simulink model "Controller_Model"  (R2015a)
settings: Solver=ode45  StartTime=0.0  StopTime=100.0  RelTol=1e-3
values from neighbouring files (symbols this model uses):
  Hph = tfest(dataPhi, [2 2], [2 2], 'Ts', Te)    [Models.m]    (also in shit_try.m = tfest(dataPhi, [2 2], [2 2], Options); smth_new_025.m = tfest(dataPhi, [6 6], [1 1], Options))
  Hphdot = tfest(dataPHId, 2, 2, 'Ts', Te)    [Models.m]    (also in shit_try.m = tfest(dataPHId, 1, 1, Options); smth_new_025.m = tfest(dataPHId, 2, 1, Options, 'Ts', Te, 'Feedthrough', true)
  Hps = tfest(dataPSI, [2 2], [1 1], 'Ts', Te)    [Models.m]    (also in shit_try.m = tfest(dataPSI, [2 2], [1 1], Options); smth_new_025.m = tfest(dataPSI, [7 7], [1 1], Options))
  Hpsdot = idtf(Hpsdot)    [Models.m]    (also in shit_try.m = tfest(dataPSdot, 1, 1, Options); smth_new_025.m = tfest(dataPSdot, 2, 2, Options, 'Ts', Te, 'Feedthrough', tru)
  Hth = tfest(dataTH, [2 2], [1 1], 'Ts', Te)    [Models.m]    (also in shit_try.m = tfest(dataTH, [2 2], [2 2], Options); smth_new_025.m = tfest(dataTH, [4 4], [4 4], Options))
  Hthdot = idtf(Hthdot)    [Models.m]    (also in shit_try.m = tfest(dataTHdot, 1, 1, Options); smth_new_025.m = tfest(dataTHdot, 2, 2, 'Ts', Te))
  K = lqr(Hf_MIMO.a, Hf_MIMO.b, Q, R)    [Models.m]    (also in shit_try.m)
  Te = t(2)-t(1)    [Models.m]    (also in shit_try.m = 0.003; simData_check.mat = 0.01; smth_new_025.m)
settings Model: Creator=Maria  LastModifiedBy=Maria

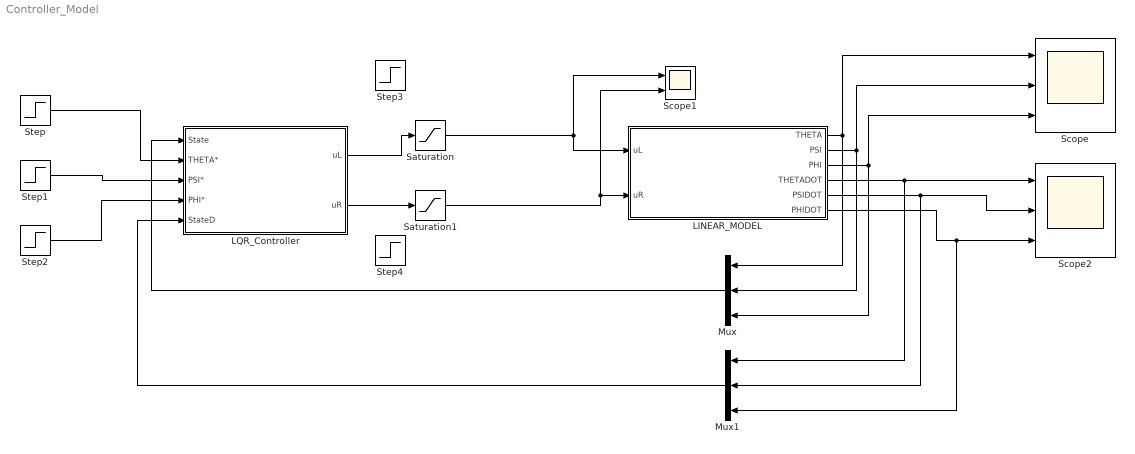
== system Controller_Model ==
  "LINEAR_MODEL " : Subsystem
  "LQR_Controller " : Subsystem
  Mux : Mux  Inputs=3
  Mux1 : Mux  Inputs=3
  Saturation : Saturate  UpperLimit=0.7  LowerLimit=-0.7
  Saturation1 : Saturate  UpperLimit=0.7  LowerLimit=-0.7
  Scope : Scope  NumInputPorts=3
      settings: YMin=-5~-5~-5  YMax=5~5~5
  Scope1 : Scope  NumInputPorts=2
      settings: YMin=-5~-5  YMax=5~5
  Scope2 : Scope  NumInputPorts=3
      settings: YMin=-5~-5~-5  YMax=5~5~5  SaveName=ScopeData2
  Step : Step  Time=0  After=0.01  SampleTime=0
  Step1 : Step  Time=0  After=0  SampleTime=0
  Step2 : Step  Time=0  After=0  SampleTime=0
  Step3 : Step  Time=0  After=0.25  SampleTime=0
  Step4 : Step  Time=0  After=0.25  SampleTime=0
  wires:
  "LINEAR_MODEL "/1("THETA ") -> Scope/1, Mux/1
  "LINEAR_MODEL "/2("PSI ") -> Mux/2, Scope/2
  "LINEAR_MODEL "/3("PHI ") -> Mux/3, Scope/3
  "LINEAR_MODEL "/4("THETADOT ") -> Mux1/1, Scope2/1
  "LINEAR_MODEL "/5("PSIDOT ") -> Scope2/2, Mux1/2
  "LINEAR_MODEL "/6("PHIDOT ") -> Mux1/3, Scope2/3
  Mux/1 -> "LQR_Controller "/1("State ")
  Step/1 -> "LQR_Controller "/2(THETA*)
  Step1/1 -> "LQR_Controller "/3("PSI* ")
  Step2/1 -> "LQR_Controller "/4("PHI* ")
  "LQR_Controller "/1("uL ") -> Saturation/1
  "LQR_Controller "/2("uR ") -> Saturation1/1
  Mux1/1 -> "LQR_Controller "/5("StateD ")
  Saturation/1 -> "LINEAR_MODEL "/1("uL "), Scope1/1
  Saturation1/1 -> Scope1/2, "LINEAR_MODEL "/2("uR ")

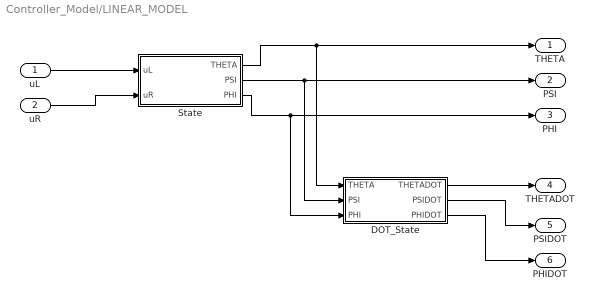
== system Controller_Model/LINEAR_MODEL  ==
  "uL " : Inport
  "uR " : Inport  Port=2
  "DOT_State " : Subsystem
  "State " : Subsystem
  "THETA " : Outport
  "PSI " : Outport  Port=2
  "PHI " : Outport  Port=3
  "THETADOT " : Outport  Port=4
  "PSIDOT " : Outport  Port=5
  "PHIDOT " : Outport  Port=6
  wires:
  "uL "/1 -> "State "/1("uL ")
  "uR "/1 -> "State "/2("uR ")
  "State "/1("THETA ") -> "THETA "/1, "DOT_State "/1("THETA ")
  "State "/2("PSI ") -> "DOT_State "/2(PSI), "PSI "/1
  "State "/3("PHI ") -> "DOT_State "/3("PHI "), "PHI "/1
  "DOT_State "/1("THETADOT ") -> "THETADOT "/1
  "DOT_State "/3("PHIDOT ") -> "PHIDOT "/1
  "DOT_State "/2("PSIDOT ") -> "PSIDOT "/1

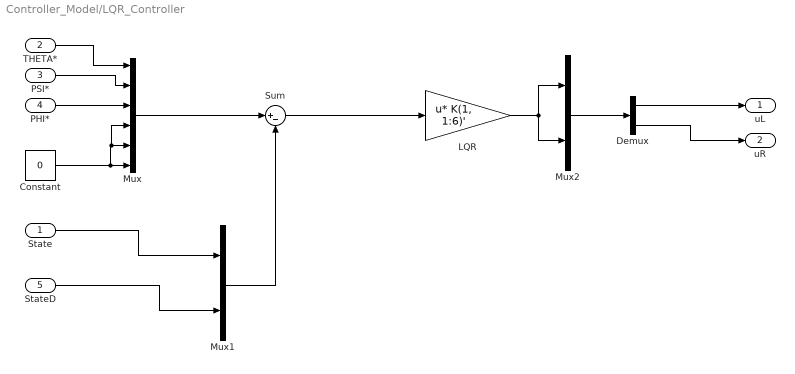
== system Controller_Model/LQR_Controller  ==
  "State " : Inport
  THETA* : Inport  Port=2
  "PSI* " : Inport  Port=3
  "PHI* " : Inport  Port=4
  "StateD " : Inport  Port=5
  Constant : Constant  Value=0
  Demux : Demux  Outputs=2
  LQR : Gain  Gain=K(1, 1:6)'  Multiplication=Matrix(u*K)
  Mux : Mux  Inputs=6
  Mux1 : Mux  Inputs=2
  Mux2 : Mux  Inputs=2
  Sum : Sum  Inputs=|+-
  "uL " : Outport
  "uR " : Outport  Port=2
  wires:
  THETA*/1 -> Mux/1
  "PSI* "/1 -> Mux/2
  "PHI* "/1 -> Mux/3
  Mux/1 -> Sum/1
  Demux/1 -> "uL "/1
  Demux/2 -> "uR "/1
  Mux1/1 -> Sum/2
  "State "/1 -> Mux1/1
  "StateD "/1 -> Mux1/2
  Constant/1 -> Mux/4, Mux/5, Mux/6
  Sum/1 -> LQR/1
  Mux2/1 -> Demux/1
  LQR/1 -> Mux2/1, Mux2/2

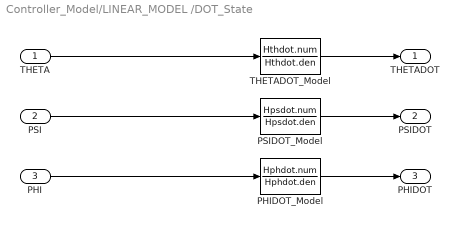
== system Controller_Model/LINEAR_MODEL /DOT_State  ==
  "THETA " : Inport
  PSI : Inport  Port=2
  "PHI " : Inport  Port=3
  "PHIDOT_Model " : DiscreteFilter  Numerator=Hphdot.num  Denominator=Hphdot.den  SampleTime=Te
  "PSIDOT_Model " : DiscreteFilter  Numerator=Hpsdot.num  Denominator=Hpsdot.den  SampleTime=Te
  "THETADOT_Model " : DiscreteFilter  Numerator=Hthdot.num  Denominator=Hthdot.den  SampleTime=Te
  "THETADOT " : Outport
  "PSIDOT " : Outport  Port=2
  "PHIDOT " : Outport  Port=3
  wires:
  "THETADOT_Model "/1 -> "THETADOT "/1
  "PSIDOT_Model "/1 -> "PSIDOT "/1
  "PHIDOT_Model "/1 -> "PHIDOT "/1
  "PHI "/1 -> "PHIDOT_Model "/1
  PSI/1 -> "PSIDOT_Model "/1
  "THETA "/1 -> "THETADOT_Model "/1

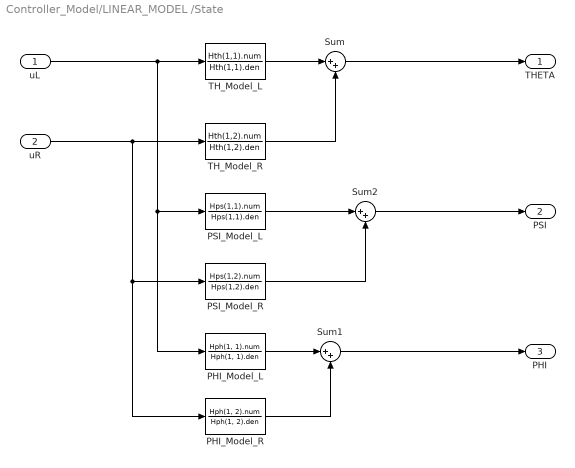
== system Controller_Model/LINEAR_MODEL /State  ==
  "uL " : Inport
  "uR " : Inport  Port=2
  "PHI_Model_L " : DiscreteFilter  Numerator=Hph(1, 1).num  Denominator=Hph(1, 1).den  SampleTime=Te
  "PHI_Model_R " : DiscreteFilter  Numerator=Hph(1, 2).num  Denominator=Hph(1, 2).den  SampleTime=Te
  "PSI_Model_L " : DiscreteFilter  Numerator=Hps(1,1).num  Denominator=Hps(1,1).den  SampleTime=Te
  "PSI_Model_R " : DiscreteFilter  Numerator=Hps(1,2).num  Denominator=Hps(1,2).den  SampleTime=Te
  Sum : Sum  Inputs=|++
  Sum1 : Sum  Inputs=|++
  Sum2 : Sum  Inputs=|++
  "TH_Model_L " : DiscreteFilter  Numerator=Hth(1,1).num  Denominator=Hth(1,1).den  SampleTime=Te
  "TH_Model_R " : DiscreteFilter  Numerator=Hth(1,2).num  Denominator=Hth(1,2).den  SampleTime=Te
  "THETA " : Outport
  "PSI " : Outport  Port=2
  "PHI " : Outport  Port=3
  wires:
  "uL "/1 -> "PSI_Model_L "/1, "PHI_Model_L "/1, "TH_Model_L "/1
  "uR "/1 -> "PSI_Model_R "/1, "PHI_Model_R "/1, "TH_Model_R "/1
  Sum/1 -> "THETA "/1
  "TH_Model_L "/1 -> Sum/1
  "TH_Model_R "/1 -> Sum/2
  "PHI_Model_L "/1 -> Sum1/1
  Sum1/1 -> "PHI "/1
  "PHI_Model_R "/1 -> Sum1/2
  "PSI_Model_L "/1 -> Sum2/1
  Sum2/1 -> "PSI "/1
  "PSI_Model_R "/1 -> Sum2/2
